simulink model "DSM_continuous"  (Simulink 7.8)
settings: Solver=ode45  StartTime=0.0  StopTime=inf  RelTol=1e-3
values from neighbouring files (symbols this model uses):
  q = [theta1;psi;theta2;y;z;]    [environment.m]
settings Model: Creator=imac  LastModifiedBy=aitor
settings SolverCC: PositivePriorityOrder=on
settings DebuggingCC: FcnCallInpInsideContextMsg=Use local settings

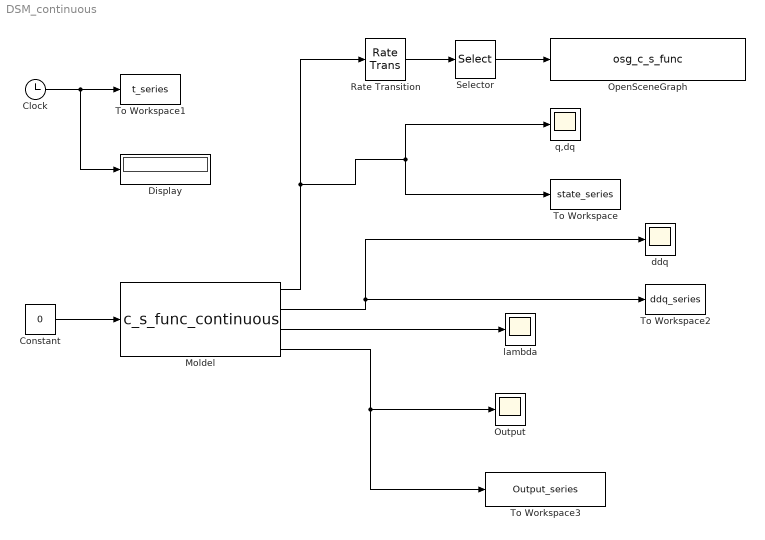
== system DSM_continuous ==
  Clock : Clock
  Constant : Constant  Value=0
  Display : Display
  Moldel : S-Function  FunctionName=c_s_func_continuous  Parameters=q dq param  EnableBusSupport=off
      mask Type: S-function: mycsfunc
      mask Description: This is a S-function that does the continuous state space system.
      mask Display: disp('[M , Phi_q''] [ddq]\n[Phi_q , 0] [lambda]\n=\n [Q ] \n   [gamma] ');
  OpenSceneGraph : S-Function  FunctionName=osg_c_s_func  EnableBusSupport=off
  Output : Scope
      settings: YMin=0  YMax=15  SaveName=ScopeData2  SampleInput=on
  Rate Transition : RateTransition  OutPortSampleTime=0.04
  Selector : Selector  InputPortWidth=2*length(q)  IndexOptions=Index vector (dialog)  Indices=1:1:length(q)  OutputSizes=1
  To Workspace : ToWorkspace  VariableName=state_series  SampleTime=-1  SaveFormat=Array
  To Workspace1 : ToWorkspace  VariableName=t_series  SampleTime=-1  SaveFormat=Array
  To Workspace2 : ToWorkspace  VariableName=ddq_series  SampleTime=-1  SaveFormat=Array
  To Workspace3 : ToWorkspace  VariableName=Output_series  SampleTime=-1  SaveFormat=Array
  ddq : Scope
      settings: YMin=-500  YMax=300  SampleInput=on
  lambda : Scope
      settings: YMin=-1750  YMax=1000  SaveName=ScopeData3  SampleInput=on
  q,dq : Scope
      settings: YMin=-0.55  YMax=0.55  SampleInput=on
  wires:
  Clock/1 -> To Workspace1/1, Display/1
  Moldel/1 -> q,dq/1, To Workspace/1, Rate Transition/1
  Moldel/2 -> To Workspace2/1, ddq/1
  Selector/1 -> OpenSceneGraph/1
  Rate Transition/1 -> Selector/1
  Moldel/4 -> Output/1, To Workspace3/1
  Moldel/3 -> lambda/1
  Constant/1 -> Moldel/1
